simulink model "PV1000_user_interface"  (R2023a)
settings: Solver=VariableStepAuto  StartTime=0.0  StopTime=100  FixedStep=0.005  RelTol=1e-3
InitFcn:
  | period = 3;
  | pulsewidth = 0.5;
  | 
  | V_T = [200 300 400 500 600];
  | Q_ref = 60*(0.001*V_T /(period*pulsewidth));
  | 
  | P_ref = [15 20 25 30 35];
libraries: instrumentlib x2, stmutilitieslib x1, slrealtimeutilitieslib x1
settings Model: Creator=Felix  LastModifiedBy=roehren
settings OptimizationCC: ReuseModelBlockBuffer=off

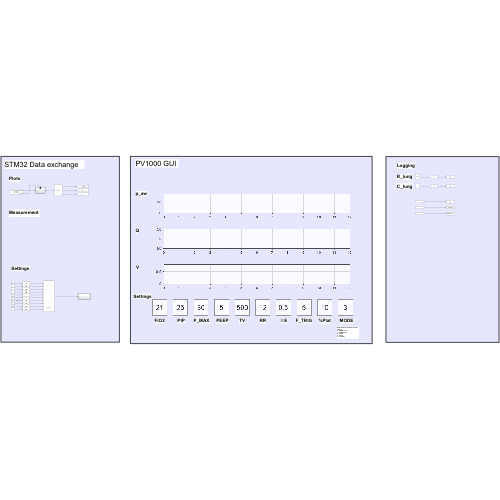
[thumbnail: Simulink's stored preview of the top-level diagram]
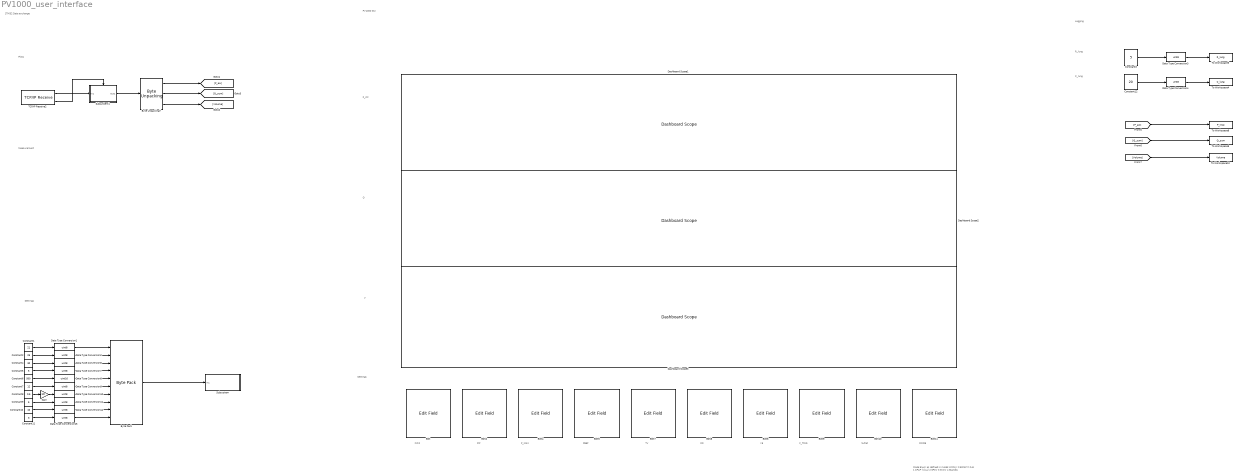
== system PV1000_user_interface ==
  note: PV1000 GUI
  note: p_aw
  note: STM32 Data exchange
  note: Plots
  note: Measurement
  note: Settings
  note: FiO2
  note: P_MAX
  note: PIP
  note: PEEP
  note: TV
  note: RR
  note: MODE
  note: %Plat
  note: I:E
  note: F_TRIG
  note: Logging
  note: R_lung
  note: C_lung
  note: Settings
  note: Q
  note: V
  note: Mode Enum as defined in model InitFcn:
      | 0 BiPAP (t.b.a)
      | 1 CPAP (t.b.a)
      | 2 SPCV
      | 3 SVCV
      | 4 Standby
  Byte Pack : stmutilitieslib/Byte Pack  datatypes={'uint8','uint8','uint8','uint8','uint16','uint8','uint8','uint8','uint8','uint8'}  byteAlign=1  blockPlatform=stm32f4discovery
  Byte Unpacking7 : slrealtimeutilitieslib/Byte Unpacking  MaskUnpackedDataTypes={'single','single','single'}  MaskUnpackedDataSizes={[1],[1],[1]}  MaskAlignment=1
  Constant1 : Constant  Value=21
  Constant10 : Constant  Value=10
  Constant11 : Constant  Value=3
  Constant12 : Constant  Value=20
  Constant2 : Constant  Value=25
  Constant3 : Constant  Value=5
  Constant4 : Constant  Value=30
  Constant5 : Constant  Value=5
  Constant6 : Constant  Value=500
  Constant7 : Constant  Value=12
  Constant8 : Constant  Value=0.5
  Constant9 : Constant  Value=5
  Dashboard Scope1 : DashboardScope  TimeSpan=12  Ymin=0  Ymax=35  ScaleAtStop=off  UpdateMode=Scroll
  Dashboard Scope2 : DashboardScope  TimeSpan=12  Ymin=-50  Ymax=50  ScaleAtStop=off  UpdateMode=Scroll
  Dashboard Scope3 : DashboardScope  TimeSpan=12  Ymin=0  Ymax=0.8  ScaleAtStop=off  UpdateMode=Scroll
  Data Type Conversion{1..4,6..7,9..11,14..15} (11 alike) : DataTypeConversion  OutDataTypeStr=uint8  SaturateOnIntegerOverflow=off  RndMeth=Floor
  Data Type Conversion8 : DataTypeConversion  OutDataTypeStr=uint16  SaturateOnIntegerOverflow=off  RndMeth=Floor
  Edit{,2,4..11} (10 alike) : EditField  LabelPosition=Hide  ShowInitialText=on  Alignment=Center
  Gain : Gain  Gain=10
  Subsystem : Subsystem  TreatAsAtomicUnit=on  SystemSampleTime=0.5
  Subsystem1 : Subsystem
  TCP/IP Receive2 : instrumentlib/TCP//IP Receive  Host=192.168.1.10  Port=25000  DataSize=[1, 12 ]  DataType=uint8  ASCIIFormatting=%f  Terminator=LF  CustomTerminator=10  ByteOrder=little-endian  EnableBlockingMode=off  Timeout=50  SampleTime=0.005  SimulateUsing=Interpreted execution
  To Workspace10 : ToWorkspace  VariableName=Volume  SaveFormat=Timeseries  SampleTime=-1
  To Workspace3 : ToWorkspace  VariableName=R_lung  SaveFormat=Timeseries  SampleTime=-1
  To Workspace4 : ToWorkspace  VariableName=C_lung  SaveFormat=Timeseries  SampleTime=-1
  To Workspace8 : ToWorkspace  VariableName=P_insp  SaveFormat=Timeseries  SampleTime=-1
  To Workspace9 : ToWorkspace  VariableName=Q_sum  SaveFormat=Timeseries  SampleTime=-1
  wires:
  Data Type Conversion1/1 -> Byte Pack/1
  Constant1/1 -> Data Type Conversion1/1
  TCP/IP Receive2/1 -> Subsystem1/1(In1)
  Constant2/1 -> Data Type Conversion2/1
  Data Type Conversion2/1 -> Byte Pack/2
  Data Type Conversion6/1 -> Byte Pack/3
  Constant4/1 -> Data Type Conversion6/1
  Data Type Conversion7/1 -> Byte Pack/4
  Data Type Conversion11/1 -> Byte Pack/8
  Constant8/1 -> Gain/1
  Data Type Conversion10/1 -> Byte Pack/7
  Data Type Conversion9/1 -> Byte Pack/6
  Constant7/1 -> Data Type Conversion9/1
  Constant6/1 -> Data Type Conversion8/1
  Data Type Conversion8/1 -> Byte Pack/5
  Constant10/1 -> Data Type Conversion14/1
  Constant11/1 -> Data Type Conversion15/1
  Data Type Conversion14/1 -> Byte Pack/9
  Data Type Conversion15/1 -> Byte Pack/10
  Constant9/1 -> Data Type Conversion11/1
  Constant5/1 -> Data Type Conversion7/1
  TCP/IP Receive2/2 -> Subsystem1/Enable
  Subsystem1/1(Out1) -> Byte Unpacking7/1
  Byte Pack/1 -> Subsystem/1(In1)
  Gain/1 -> Data Type Conversion10/1
  Constant3/1 -> Data Type Conversion3/1
  Data Type Conversion3/1 -> To Workspace3/1
  Data Type Conversion4/1 -> To Workspace4/1
  Constant12/1 -> Data Type Conversion4/1
  [P_aw] -> To Workspace8/1
  [Q_sum] -> To Workspace9/1
  [Volume] -> To Workspace10/1
  Byte Unpacking7/1 -> [P_aw]
  Byte Unpacking7/2 -> [Q_sum]
  Byte Unpacking7/3 -> [Volume]

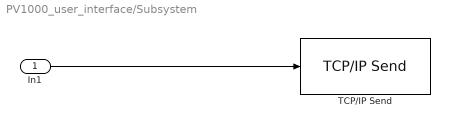
== system PV1000_user_interface/Subsystem ==
  In1 : Inport
  TCP/IP Send : instrumentlib/TCP//IP Send  Host=192.168.1.10  Port=25005  ByteOrder=little-endian  EnableBlockingMode=on  Timeout=10  TransferDelay=on  SimulateUsing=Interpreted execution
  wires:
  In1/1 -> TCP/IP Send/1

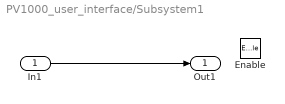
== system PV1000_user_interface/Subsystem1 ==
  In1 : Inport
  Enable : EnablePort
  Out1 : Outport
  wires:
  In1/1 -> Out1/1
